simulink model "BD_PAR_AUTO_base_model"  (Simulink 10.3)
settings: Solver=ode1  StartTime=0.0  StopTime=max(cyc_mph(:,1))  FixedStep=1  MaxStep=1  RelTol=1e-3  AbsTol=1e-3
undefined symbols (not defined in the file): acc_dcdc_eff, acc_elec_eff, acc_elec_pwr, acc_mech_eff, acc_mech_pwr, acc_mech_trq, air_cp, amb_tmp, cs_charge_deplete_bool, cs_charge_trq, cs_electric_decel_spd, cs_electric_launch_spd_hi, cs_electric_launch_spd_lo, cs_hi_soc, cs_lo_soc, cs_min_trq_frac, cs_off_trq_frac, cyc_avg_time, cyc_cargo_mass, cyc_elevation_init, cyc_filter_bool, cyc_grade, cyc_mph, enable_sim_stop_distance, enable_sim_stop_max_spd, enable_sim_stop_speed, enable_sim_stop_time, enable_stop, enable_stop_fc, ess_cap_scale, ess_coulombic_eff, ess_init_soc, ess_max_ah_cap, ess_max_volts, ess_min_volts, ess_mod_airflow, ess_mod_cp, ess_mod_init_tmp, ess_module_mass, ess_module_num, ess_on, ess_r_chg, ess_r_dis, ess_res_scale_coef, ess_res_scale_fun, ess_set_tmp, ess_soc, ess_th_calc, ess_th_res_off, ess_th_res_on, ess_tmp, ess_voc, ex_calc, ex_cat_co_frac, ex_cat_ext_cp, ex_cat_ext_emisv, ex_cat_ext_init_tmp, ex_cat_ext_mass, ex_cat_ext_sarea, ex_cat_hc_frac ... (+168)
(part 4 of 15)

== system BD_PAR_AUTO_base_model/hydraulic torque converter for  parallel hybrid <htc>/effect of inertia (Nm) ==
  note: This block computes the torque required to overcome the inertia of the
      | turbine (plus 1/2 fluid in htc).
  turbine/output speed (rad/s) : Inport
  Constant : Constant  Value=htc_inertia
  Product : Product  SaturateOnIntegerOverflow=on
  d/dt : Derivative
  inertia torque (Nm) : Outport  InitialOutput=0
  wires:
  d/dt/1 -> Product/1
  turbine/output speed (rad/s)/1 -> d/dt/1
  Constant/1 -> Product/2
  Product/1 -> inertia torque (Nm)/1

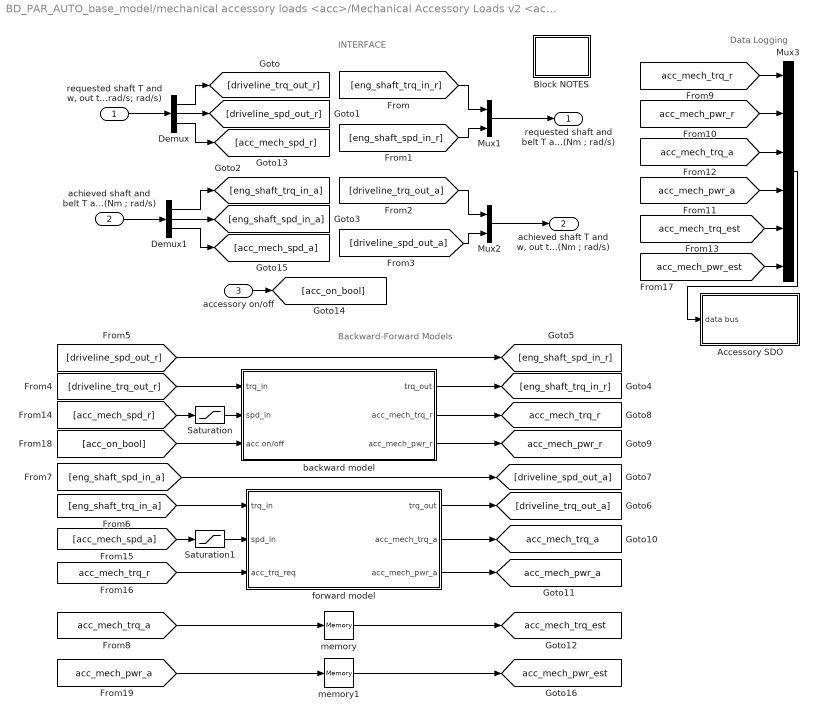
== system BD_PAR_AUTO_base_model/mechanical accessory loads <acc>/Mechanical Accessory Loads v2 <acc> ==
  note: Data Logging
  note: Backward-Forward Models
  note: INTERFACE
  "requested shaft T and w, out to the driveline  (Nm ; rad/s; rad/s)" : Inport
  "achieved shaft and belt T and w, in from the prime mover (Nm ; rad/s)" : Inport  Port=2
  accessory on/off : Inport  Port=3
  Accessory SDO : Subsystem
  Block NOTES : Subsystem
      mask Display: disp('Block\nNOTES')
  Demux : Demux  Outputs=3
      settings: DisplayOption=none
  Demux1 : Demux  Outputs=3
      settings: DisplayOption=none
  Mux1 : Mux  Inputs=2
  Mux2 : Mux  Inputs=2
  Mux3 : Mux  Inputs=6
  Saturation : Saturate  UpperLimit=acc_max_spd  LowerLimit=acc_min_spd
  Saturation1 : Saturate  UpperLimit=acc_max_spd  LowerLimit=acc_min_spd
  backward model : Subsystem
  forward model : Subsystem
  memory : Memory  InitialCondition=ic_mech_trq
  memory1 : Memory  InitialCondition=ic_mech_pwr
  "requested shaft and belt T and w, in from the prime mover (Nm ; rad/s)" : Outport
  "achieved shaft T and w, out to the driveline (Nm ; rad/s)" : Outport  Port=2
  tag scope: acc_mech_pwr_a=global, acc_mech_pwr_est=global, acc_mech_pwr_r=global, acc_mech_trq_a=global, acc_mech_trq_est=global, acc_mech_trq_r=global
  wires:
  [acc_mech_pwr_a] -> memory1/1
  [acc_mech_trq_a] -> memory/1
  memory1/1 -> [acc_mech_pwr_est]
  memory/1 -> [acc_mech_trq_est]
  [acc_mech_pwr_est] -> Mux3/6
  Demux/3 -> [acc_mech_spd_r]
  Demux1/3 -> [acc_mech_spd_a]
  [acc_mech_trq_r] -> forward model/3(acc_trq_req)
  Saturation/1 -> backward model/2(spd_in)
  [acc_mech_spd_r] -> Saturation/1
  Saturation1/1 -> forward model/2(spd_in)
  [acc_mech_spd_a] -> Saturation1/1
  forward model/3(acc_mech_pwr_a) -> [acc_mech_pwr_a]
  forward model/2(acc_mech_trq_a) -> [acc_mech_trq_a]
  forward model/1(trq_out) -> [driveline_trq_out_a]
  [acc_on_bool] -> backward model/3(acc on/off)
  accessory on/off/1 -> [acc_on_bool]
  [eng_shaft_trq_in_a] -> forward model/1(trq_in)
  [acc_mech_pwr_a] -> Mux3/4
  [acc_mech_trq_a] -> Mux3/3
  [eng_shaft_spd_in_a] -> [driveline_spd_out_a]
  [driveline_spd_out_r] -> [eng_shaft_spd_in_r]
  [acc_mech_trq_est] -> Mux3/5
  Mux3/1 -> Accessory SDO/1(data bus)
  [acc_mech_pwr_r] -> Mux3/2
  [acc_mech_trq_r] -> Mux3/1
  backward model/1(trq_out) -> [eng_shaft_trq_in_r]
  [driveline_trq_out_r] -> backward model/1(trq_in)
  backward model/3(acc_mech_pwr_r) -> [acc_mech_pwr_r]
  backward model/2(acc_mech_trq_r) -> [acc_mech_trq_r]
  [driveline_spd_out_a] -> Mux2/2
  [driveline_trq_out_a] -> Mux2/1
  Mux2/1 -> "achieved shaft T and w, out to the driveline (Nm ; rad/s)"/1
  [eng_shaft_spd_in_r] -> Mux1/2
  [eng_shaft_trq_in_r] -> Mux1/1
  Mux1/1 -> "requested shaft and belt T and w, in from the prime mover (Nm ; rad/s)"/1
  Demux1/2 -> [eng_shaft_spd_in_a]
  Demux1/1 -> [eng_shaft_trq_in_a]
  "achieved shaft and belt T and w, in from the prime mover (Nm ; rad/s)"/1 -> Demux1/1
  Demux/2 -> [driveline_spd_out_r]
  Demux/1 -> [driveline_trq_out_r]
  "requested shaft T and w, out to the driveline  (Nm ; rad/s; rad/s)"/1 -> Demux/1

== system BD_PAR_AUTO_base_model/motor/ controller <mc> par/Block NOTES ==
  note: Available torque is computed from available power by assuming that the ratio of rotor torque to input
      | (electric) power is the same for the actual/achievable situation as was computed for the request.  This
      | is mathematically equivalent to assuming that the motor/controller efficiency.  Rotor speed for the
      | actual/achievable calculations is as computed in the 'request' branch.
  note: This motor/controller model includes loss data, rotational inertia, and performance limits.

== system BD_PAR_AUTO_base_model/motor/ controller <mc> par/N-m drive torque per W input ==
  req'd input power (W) : Inport
  req'd rotor drive torque (Nm) : Inport  Port=2
  Block NOTES : Subsystem
      mask Display: disp('Block\nNOTES')
  Constant : Constant  Value=eps
  Constant1 : Constant  Value=0
  Constant2 : Constant  Value=inf
  Product : Product  Inputs=/*  SaturateOnIntegerOverflow=on
  Relational Operator : RelationalOperator  Operator=~=  RndMeth=Nearest  InputSameDT=on
  Sum : Sum  SaturateOnIntegerOverflow=on
  Switch : Switch  Threshold=eps
  Nm per W : Outport  InitialOutput=0
  wires:
  Constant2/1 -> Switch/3
  Constant1/1 -> Relational Operator/2
  req'd input power (W)/1 -> Relational Operator/1, Sum/2
  Sum/1 -> Product/1
  Switch/1 -> Nm per W/1
  Relational Operator/1 -> Switch/2
  Product/1 -> Switch/1
  req'd rotor drive torque (Nm)/1 -> Product/2
  Constant/1 -> Sum/1

== system BD_PAR_AUTO_base_model/motor/ controller <mc> par/documentation10 ==

== system BD_PAR_AUTO_base_model/motor/ controller <mc> par/effect of inertia (Nm) ==
  mc_spd_out_a : Inport
  Block NOTES : Subsystem
      mask Display: disp('Block\nNOTES')
  Constant : Constant  Value=eps
  Constant1 : Constant  Value=max(mc_max_trq)*mc_trq_scale*mc_overtrq_factor
  Constant2 : Constant  Value=gb_ratio(1)*fd_ratio/wh_radius
  Gain : Gain  Gain=mc_inertia  SaturateOnIntegerOverflow=on
  Memory : Memory
  MinMax : MinMax  Inputs=2
  Product : Product  SaturateOnIntegerOverflow=on
  Sum : Sum  SaturateOnIntegerOverflow=on
  Switch : Switch  Threshold=eps
  alpha : Derivative
  motor inertia as a function of total vehicle inertia (generous approximation) : Subsystem
  overall gear ratio / wh_radius : Product  Inputs=*/  SaturateOnIntegerOverflow=on
  out_1 : Outport  InitialOutput=0
  wires:
  Switch/1 -> overall gear ratio / wh_radius/2
  Constant2/1 -> Switch/3
  [veh_spd_a_rec] -> Switch/2, Sum/1
  Sum/1 -> Switch/1
  Constant/1 -> Sum/2
  motor inertia as a function of total vehicle inertia (generous approximation)/1(Out1) -> Product/2
  Memory/1 -> motor inertia as a function of total vehicle inertia (generous approximation)/1(gear ratio)
  Constant1/1 -> Product/1
  overall gear ratio / wh_radius/1 -> Memory/1
  Product/1 -> MinMax/2
  Gain/1 -> MinMax/1
  MinMax/1 -> out_1/1
  mc_spd_out_a/1 -> overall gear ratio / wh_radius/1, alpha/1
  alpha/1 -> Gain/1

== system BD_PAR_AUTO_base_model/motor/ controller <mc> par/enforce torque limit ==
  req'd motor torque (Nm) : Inport
  limited motor speed (rad/s) : Inport  Port=2
  Block NOTES : Subsystem
      mask Display: disp('Block\nNOTES')
  MinMax : MinMax  Inputs=2
  MinMax1 : MinMax  Function=max  Inputs=2
  Relational Operator2 : RelationalOperator  Operator=~=  RndMeth=Nearest  InputSameDT=on
  Switch : Switch
  To WS2 : ToWorkspace  VariableName=mc_max_trq_vec
      settings: MaxDataPoints=50000
  max gen torque : Lookup  InputValues=mc_map_spd*mc_spd_scale  Table=mc_max_gen_trq*mc_overtrq_factor*mc_trq_scale
  max torque : Lookup  InputValues=mc_map_spd*mc_spd_scale  Table=mc_max_trq*mc_overtrq_factor*mc_trq_scale
  limited motor torque (Nm) : Outport
  tag scope: mc_trq_limited=global
  wires:
  max gen torque/1 -> MinMax1/2
  limited motor speed (rad/s)/1 -> max gen torque/1, max torque/1
  Relational Operator2/1 -> [mc_trq_limited]
  MinMax/1 -> Switch/1
  MinMax1/1 -> Switch/3
  Switch/1 -> limited motor torque (Nm)/1, Relational Operator2/2
  req'd motor torque (Nm)/1 -> MinMax/1, MinMax1/1, Switch/2, Relational Operator2/1
  max torque/1 -> MinMax/2, To WS2/1

== system BD_PAR_AUTO_base_model/motor/ controller <mc> par/mc tmp ==
  Qmc_gen : Inport
  veh spd : Inport  Port=2
  key ON? : Inport  Port=3
  Enable : EnablePort  StatesWhenEnabling=reset
  1/mcp : Gain  Gain=1/(mc_mass*mc_cp)  SaturateOnIntegerOverflow=on
  >=0 : Saturate  UpperLimit=Inf  LowerLimit=0
  ">=0 " : Saturate  UpperLimit=Inf  LowerLimit=0
  Block NOTES : Subsystem
      mask Display: disp('Block\nNOTES')
  Mux10 : Mux  Inputs=2
  Mux9 : Mux  Inputs=2
  Qa : Fcn  Expr=u(1)*(mc_sarea*mc_trq_scale*mc_spd_scale)*u(2)
  Qc1 : Sum  Inputs=-+  SaturateOnIntegerOverflow=on
  Qnet : Sum  Inputs=+++  SaturateOnIntegerOverflow=on
  Qp2a,v7 : Fcn  Expr=amb_tmp-u(1)
  Qr : Fcn  Expr=0.9*(5.67e-8)*(mc_sarea*mc_trq_scale*mc_spd_scale)*((amb_tmp+273)^4 - (u(1)+273)^4)
  Tmc3 : Integrator  InitialCondition=mc_init_tmp
  Va/Vv : Gain  Gain=0.5  SaturateOnIntegerOverflow=on
  ha : Fcn  Expr=6 + 6*((abs(u(2))/1000))^0.25 + 60*(abs(u(1))/30)^0.63
  mc coolant : Subsystem  TreatAsAtomicUnit=on
  Tmc : Outport  InitialOutput=0
  Qmc_clt : Outport  Port=2  OutputWhenDisabled=reset  InitialOutput=0
  wires:
  Qnet/1 -> Qc1/2, mc coolant/2("Qmc ")
  Qc1/1 -> 1/mcp/1
  1/mcp/1 -> Tmc3/1
  Tmc3/1 -> Qp2a,v7/1, Qr/1, Tmc/1, mc coolant/1(Tcl)
  mc coolant/1(Qmc_clt) -> Qc1/1, >=0/1
  >=0/1 -> Qmc_clt/1
  key ON?/1 -> mc coolant/Enable
  veh spd/1 -> Va/Vv/1
  Qa/1 -> Qnet/2
  ">=0 "/1 -> Qnet/1
  Qmc_gen/1 -> ">=0 "/1
  Qr/1 -> Qnet/3
  Qp2a,v7/1 -> Mux10/2, Mux9/2
  ha/1 -> Mux10/1
  Va/Vv/1 -> Mux9/1
  Mux9/1 -> ha/1
  Mux10/1 -> Qa/1

== system BD_PAR_AUTO_base_model/motor/ controller <mc> par/motor controller logic interface ==
  w_mc_out_r : Inport
  P_mc_in_1lim : Inport  Port=2
  P_mc_in_r : Outport  InitialOutput=0
  tag scope: P_mc_in_1lim=global, w_mc_out_r=global
  wires:
  [P_mc_in_r] -> P_mc_in_r/1
  w_mc_out_r/1 -> [w_mc_out_r]
  P_mc_in_1lim/1 -> [P_mc_in_1lim]

== system BD_PAR_AUTO_base_model/motor/ controller <mc> par/motor speed estimator ==
  mc_spd_out_a : Inport
  <= max spd : Saturate  UpperLimit=max(mc_map_spd)*mc_spd_scale  LowerLimit=-inf
  Block NOTES : Subsystem
      mask Display: disp('Block\nNOTES')
  Constant : Constant  Value=eps
  Constant1 : Constant  Value=0
  Constant2 : Constant  Value=2
  Gain : Gain  Gain=0.447  SaturateOnIntegerOverflow=on
  Logical Operator1 : Logic
  Memory : Memory  InitialCondition=cyc_mph(1,2)*0.447/wh_radius*fd_ratio*max(gb_ratio)*tc_mc_to_fc_ratio
  Memory1 : Memory  InitialCondition=1
  Memory2 : Memory
  Product : Product  Inputs=**/  SaturateOnIntegerOverflow=on
  Relational : RelationalOperator  Operator=>  RndMeth=Nearest  InputSameDT=on
  Relational Operator1 : RelationalOperator  Operator=~=  RndMeth=Nearest  InputSameDT=on
  Sum : Sum  SaturateOnIntegerOverflow=on
  Sum1 : Sum  Inputs=-+  SaturateOnIntegerOverflow=on
  Switch : Switch  Threshold=eps
  Switch1 : Switch  Threshold=eps
  To Workspace7 : ToWorkspace  VariableName=mc_spd_est  SampleTime=-1
  Out1 : Outport
  tag scope: mc_spd_limited=global
  wires:
  Switch/1 -> Memory/1
  Memory1/1 -> Switch1/2
  Relational/1 -> Memory1/1
  Sum1/1 -> Relational/1
  Constant2/1 -> Relational/2
  [mpha] -> Sum1/1, Gain/1
  [cyc_mph_r] -> Sum1/2
  Constant/1 -> Sum/2
  Memory/1 -> Switch1/1
  Constant1/1 -> Switch/3
  [veh_spd_a_rec] -> Switch/2, Sum/1
  Gain/1 -> Product/2
  Sum/1 -> Product/3
  Product/1 -> Switch/1
  mc_spd_out_a/1 -> Product/1, Switch1/3
  Memory2/1 -> Logical Operator1/2
  Logical Operator1/1 -> [mc_spd_limited]
  Relational Operator1/1 -> Logical Operator1/1, Memory2/1
  Switch1/1 -> <= max spd/1, Relational Operator1/1
  <= max spd/1 -> Out1/1, To Workspace7/1, Relational Operator1/2

== system BD_PAR_AUTO_base_model/motor/ controller <mc> par/rotor drive torque available (Nm) ==
  torque per unit input power (N-m/W) : Inport
  available input power (W) : Inport  Port=2
  Block NOTES : Subsystem
      mask Display: disp('Block\nNOTES')
  Constant2 : Constant  Value=inf
  Constant3 : Constant  Value=0
  Product : Product  SaturateOnIntegerOverflow=on
  Relational Operator : RelationalOperator  Operator=~=  RndMeth=Nearest  InputSameDT=on
  Switch : Switch  Threshold=eps
  rotor drive torque available : Outport  InitialOutput=0
  wires:
  torque per unit input power (N-m/W)/1 -> Relational Operator/1, Product/1
  Switch/1 -> rotor drive torque available/1
  Relational Operator/1 -> Switch/2
  Product/1 -> Switch/1
  available input power (W)/1 -> Product/2
  Constant2/1 -> Relational Operator/2
  Constant3/1 -> Switch/3

== system BD_PAR_AUTO_base_model/power bus <pb>/Block NOTES ==
  note: This power bus requires power from (or distributes power to)
      | the generator first, taking the balance from the energy
      | storage system.

== system BD_PAR_AUTO_base_model/torque coupler <tc>/Block NOTES ==
  note: speed, while the motor's speed may be different.  The ratio of motor speed to main
      | output speed is stored in the variable tc_mc_to_fc_spd_ratio.
  note: This block models a chain- or belt-driven torque coupler, with three gears:  one each
      | for the motor, main input (the engine or gearbox), and main output (to the gearbox
      | or final drive).  It includes losses in the chain or belt, but leaves inertia effects to be
      | considered in the appropriate component.
      |
      | The entire torque required out of the torque coupler (plus losses) is required from the
      | engine.  The engine provides only as much torque as its engine controller (see the
      | <vc> block) allows.  Any remaining unmet torque request is submitted to the motor,
      | which meets the request to the best of its ability.
      |
      | The torque converter output speed is limited by the maximum speeds of both the
      | motor and the engine.
      |
      | The loss torque is zero when the gears are not turning, and is applied at the output
      |  gear.
      |
      | The gears connecting the main input and main output to the torque converter's belt
      | or chain are assumed to be of the same size, so that main input speed = main output

== system BD_PAR_AUTO_base_model/torque coupler <tc>/help ==

== system BD_PAR_AUTO_base_model/torque coupler <tc>/loss (Nm) ==
  note: The loss torque is zero when the gears are not turning,
      | and is applied at the torque coupler's output gear.
  tc output speed (rad/s) : Inport
  Constant : Constant  Value=0
  Switch : Switch  Threshold=eps
  torque coupler loss torque (Nm) : Constant  Value=tc_loss
  drag torque (Nm) : Outport  InitialOutput=0
  wires:
  torque coupler loss torque (Nm)/1 -> Switch/1
  Switch/1 -> drag torque (Nm)/1
  tc output speed (rad/s)/1 -> Switch/2
  Constant/1 -> Switch/3

== system BD_PAR_AUTO_base_model/vehicle <veh>/Block NOTES ==
  note: A slight simplification, the assumption that (speed_at_end_of_time_step)^2 is roughly equal to
      | (speed_at_end_of_time_step)*(speed_at_beginning_of_time_step), is used to avoid solving
      | a quadratic equation in the solution of v=v(Ftract).
  note: This block uses the required vehicle speed with vehicle parameters and the previous speed
      | and classic, straightforward equations to determine the tractive force required at the tire/road interface.
  note: If no drivetrain component ran up against its performance limit during the time step, the achieved speed
      | is taken to be the requested speed.
  note: Given the tractive force available, this block uses the same equations to determine the achievable speed.

== system BD_PAR_AUTO_base_model/vehicle <veh>/force req'd to accelerate (N) ==
  v(m/s) : Inport
  v prev : Inport  Port=2
  Clock : Clock
  Memory : Memory  InitialCondition=-0.1
  Product1 : Product  Inputs=**/  SaturateOnIntegerOverflow=on
  Sum : Sum  Inputs=+-  SaturateOnIntegerOverflow=on
  Sum1 : Sum  Inputs=+-  SaturateOnIntegerOverflow=on
  current veh mass : Subsystem
  (N) : Outport  InitialOutput=0
  wires:
  current veh mass/1(Out1) -> Product1/1
  Clock/1 -> Sum1/1, Memory/1
  Memory/1 -> Sum1/2
  Product1/1 -> (N)/1
  v prev/1 -> Sum/2
  v(m/s)/1 -> Sum/1
  Sum1/1 -> Product1/3
  Sum/1 -> Product1/2

== system BD_PAR_AUTO_base_model/vehicle <veh>/force req'd to ascend (N) ==
  average vehicle speed over time step (m/s) : Inport
  Constant : Constant  Value=veh_gravity
  Constant1 : Constant  Value=0
  Product : Product  Inputs=3  SaturateOnIntegerOverflow=on
  Switch : Switch
  Trigonometric Function : Trigonometry  Operator=atan
  Trigonometric Function1 : Trigonometry
  current veh mass : Subsystem
  (N) : Outport  InitialOutput=0
  wires:
  current veh mass/1(Out1) -> Product/3
  average vehicle speed over time step (m/s)/1 -> Switch/2
  Constant1/1 -> Switch/3
  Switch/1 -> (N)/1
  Product/1 -> Switch/1
  Constant/1 -> Product/1
  [grade] -> Trigonometric Function/1
  Trigonometric Function1/1 -> Product/2
  Trigonometric Function/1 -> Trigonometric Function1/1

== system BD_PAR_AUTO_base_model/vehicle <veh>/force req'd to overcome aerodynamic drag (N) ==
  average vehicle speed over time step (m/s) : Inport
  Constant : Constant  Value=veh_air_density*veh_CD*veh_FA*0.5
  Product : Product  Inputs=3  SaturateOnIntegerOverflow=on
  D aero(N) : Outport  InitialOutput=0
  wires:
  Product/1 -> D aero(N)/1
  Constant/1 -> Product/3
  average vehicle speed over time step (m/s)/1 -> Product/2, Product/1

== system BD_PAR_AUTO_base_model/vehicle <veh>/help ==

== system BD_PAR_AUTO_base_model/vehicle <veh>/record achieved force outputs ==
  spd_prev : Inport
  spd : Inport  Port=2
  Gain1 : Gain  Gain=0.5  SaturateOnIntegerOverflow=on
  Product{,1..3} (4 alike) : Product  SaturateOnIntegerOverflow=on
  Sum2 : Sum  SaturateOnIntegerOverflow=on
  To Workspace1 : ToWorkspace  VariableName=veh_pwr_rr_a  SampleTime=-1
  To Workspace4 : ToWorkspace  VariableName=veh_pwr_accel_a  SampleTime=-1
  To Workspace6 : ToWorkspace  VariableName=veh_pwr_drag_a  SampleTime=-1
  To Workspace7 : ToWorkspace  VariableName=veh_pwr_ascent_a  SampleTime=-1
  force req'd to accelerate (N)1 : Subsystem
  force req'd to ascend (N)1 : Subsystem
  force req'd to overcome aerodynamic drag (N)1 : Subsystem
  rolling resistance force : Subsystem  BlockChoice=force req'd to overcome rolling resistance (N)
      settings: AttributesFormatString=%<BlockChoice>  TemplateBlock=lib_vehicle/Submodels/rolling resistance force  MemberBlocks=force req'd to overcome rolling resistance (N),force req'd to overcome rolling resistance (N) j2452
  tag scope: veh_pwr_accel_a=global, veh_pwr_ascent_a=global, veh_pwr_drag_a=global, veh_pwr_rr_a=global
  wires:
  Gain1/1 -> [vel_ave], rolling resistance force/1(average vehicle speed over time step (m/s)), force req'd to ascend (N)1/1(average vehicle speed over time step (m/s)), force req'd to overcome aerodynamic drag (N)1/1(average vehicle speed over time step (m/s))
  Product3/1 -> To Workspace1/1, [veh_pwr_rr_a]
  [vel_ave] -> Product3/2
  Product2/1 -> [veh_pwr_ascent_a], To Workspace7/1
  [vel_ave] -> Product2/2
  [vel_ave] -> Product1/2
  [vel_ave] -> Product/2
  Product1/1 -> [veh_pwr_drag_a], To Workspace6/1
  Product/1 -> [veh_pwr_accel_a], To Workspace4/1
  force req'd to accelerate (N)1/1((N)) -> Product/1
  rolling resistance force/1(Fr (N)) -> Product3/1
  force req'd to ascend (N)1/1((N)) -> Product2/1
  force req'd to overcome aerodynamic drag (N)1/1(D aero(N)) -> Product1/1
  spd_prev/1 -> Sum2/2, force req'd to accelerate (N)1/2(v prev)
  spd/1 -> Sum2/1, force req'd to accelerate (N)1/1(v(m/s))
  Sum2/1 -> Gain1/1

== system BD_PAR_AUTO_base_model/vehicle <veh>/rolling resistance force ==
  average vehicle speed over time step (m/s) : Inport
  force req'd to overcome rolling resistance (N) : Subsystem
  Fr (N) : Outport
  wires:
  average vehicle speed over time step (m/s)/1 -> force req'd to overcome rolling resistance (N)/1(average vehicle speed over time step (m/s))
  force req'd to overcome rolling resistance (N)/1(Fr (N)) -> Fr (N)/1

== system BD_PAR_AUTO_base_model/vehicle <veh>/vehicle speed ==
  vehicle speed at beginning of time step (m/s) : Inport
  "available tractive force and linear speed (N), (m/s)" : Inport  Port=2
  vehicle speed (m/s) : Subsystem
  vehicle speed achievable at end of time step (m/s) : Outport
  wires:
  vehicle speed at beginning of time step (m/s)/1 -> vehicle speed (m/s)/1(vehicle speed at beginning of time step (m/s))
  "available tractive force and linear speed (N), (m/s)"/1 -> vehicle speed (m/s)/2("available tractive force and linear speed (N), (m/s)")
  vehicle speed (m/s)/1(vehicle speed achievable at end of time step (m/s)) -> vehicle speed achievable at end of time step (m/s)/1

== system BD_PAR_AUTO_base_model/wheel and axle  front/rear <wh>/Block NOTES ==
  note: This block determines the required axle torque and speed given the tractive force and
      | speed required to meet the trace in the top blocks, and determines the available tractive
      | force and possible vehicle speed given the drivetrain-input torque and rotational speed
      | in the bottom blocks.  The "wheel control" blocks apply the braking strategy and ensure
      | that accelerations beyond the capability of the tires are not requested.

== system BD_PAR_AUTO_base_model/wheel and axle  front/rear <wh>/effect of  inertia (Nm) ==
  note: This block computes the torque required to overcome the inertia of the
      | wheels and axle.
  axle input speed (rad/s) : Inport
  Constant : Constant  Value=wh_inertia
  Product : Product  SaturateOnIntegerOverflow=on
  d/dt : Derivative
  inertia torque (Nm) : Outport  InitialOutput=0
  wires:
  Product/1 -> inertia torque (Nm)/1
  Constant/1 -> Product/2
  axle input speed (rad/s)/1 -> d/dt/1
  d/dt/1 -> Product/1

== system BD_PAR_AUTO_base_model/wheel and axle  front/rear <wh>/front brake ==
  F_brake : Inport
  Constant : Constant  Value=wh_max_front_brake_force
  Terminator : Terminator
  F_brake_max : Outport  InitialOutput=0
  wires:
  Constant/1 -> F_brake_max/1
  F_brake/1 -> Terminator/1

== system BD_PAR_AUTO_base_model/wheel and axle  front/rear <wh>/front force ==
  In1 : Inport
  In2 : Inport  Port=2
  Product1 : Product  SaturateOnIntegerOverflow=on
  Sum2 : Sum  Inputs=-+  SaturateOnIntegerOverflow=on
  To Workspace12 : ToWorkspace  VariableName=wh_front_brake_r  SampleTime=-1
  brake request  controller interface : Subsystem
  tractive torque req/d of drivetrain (Nm) : Gain  Gain=wh_radius  SaturateOnIntegerOverflow=on
  Out1 : Outport
  wires:
  tractive torque req/d of drivetrain (Nm)/1 -> Out1/1
  In2/1 -> Product1/2
  In1/1 -> Product1/1
  Product1/1 -> Sum2/2
  Sum2/1 -> tractive torque req/d of drivetrain (Nm)/1
  brake request  controller interface/1(F_front_brake_req) -> To Workspace12/1, Sum2/1

== system BD_PAR_AUTO_base_model/wheel and axle  front/rear <wh>/front/rear brake controller interface (achievable) ==
  F_drivetrain_ach : Inport
  w_wheel_ach : Inport  Port=2
  F_rear_drivetrain_ach : Inport  Port=3
  F_max_front_brake : Inport  Port=4
  F_max_rear_brake : Inport  Port=5
  F_front_brake : Outport  InitialOutput=0
  F_rear_brake : Outport  Port=2  InitialOutput=0
  tag scope: F_drivetrain_ach=global, F_max_front_brake=global, F_max_rear_brake=global, F_rear_drivetrain_ach=global, w_wheel_ach=global
  wires:
  F_rear_drivetrain_ach/1 -> [F_rear_drivetrain_ach]
  F_max_rear_brake/1 -> [F_max_rear_brake]
  F_max_front_brake/1 -> [F_max_front_brake]
  F_drivetrain_ach/1 -> [F_drivetrain_ach]
  w_wheel_ach/1 -> [w_wheel_ach]
  [F_front_brake] -> F_front_brake/1
  [F_rear_brake] -> F_rear_brake/1

== system BD_PAR_AUTO_base_model/wheel and axle  front/rear <wh>/help ==

== system BD_PAR_AUTO_base_model/wheel and axle  front/rear <wh>/limits and losses diagnostics ==
  speed : Inport
  front brake : Inport  Port=2
  front brake max : Inport  Port=3
  rear brake max : Inport  Port=4
  rear brake : Inport  Port=5
  Gain : Gain  Gain=-1  SaturateOnIntegerOverflow=on
  Logical Operator : Logic  Operator=OR
  Product : Product  SaturateOnIntegerOverflow=on
  Relational Operator1 : RelationalOperator  Operator===  RndMeth=Nearest  InputSameDT=on
  Relational Operator2 : RelationalOperator  Operator===  RndMeth=Nearest  InputSameDT=on
  Sum3 : Sum  SaturateOnIntegerOverflow=on
  To Workspace6 : ToWorkspace  VariableName=wh_brake_loss_pwr  SampleTime=-1
  tag scope: brake_limited=global
  wires:
  rear brake/1 -> Relational Operator2/2, Sum3/2
  rear brake max/1 -> Relational Operator2/1
  front brake max/1 -> Relational Operator1/2
  front brake/1 -> Relational Operator1/1, Sum3/1
  speed/1 -> Product/1
  Relational Operator2/1 -> Logical Operator/2
  Relational Operator1/1 -> Logical Operator/1
  Logical Operator/1 -> [brake_limited]
  Product/1 -> To Workspace6/1
  Sum3/1 -> Gain/1
  Gain/1 -> Product/2

== system BD_PAR_AUTO_base_model/wheel and axle  front/rear <wh>/loss (Nm) ==
  note: The loss torque is zero when the axle is not turning.
  axle speed (rad/s) : Inport
  Constant : Constant  Value=0
  Switch : Switch  Threshold=eps
  veh mass calc : Subsystem
  wheel & axle bearing drag (Nm) : Lookup  InputValues=wh_axle_loss_mass  Table=wh_axle_loss_trq
  drag torque (Nm) : Outport  InitialOutput=0
  wires:
  wheel & axle bearing drag (Nm)/1 -> Switch/1
  Constant/1 -> Switch/3
  axle speed (rad/s)/1 -> Switch/2
  Switch/1 -> drag torque (Nm)/1
  veh mass calc/1(Out1) -> wheel & axle bearing drag (Nm)/1

== system BD_PAR_AUTO_base_model/wheel and axle  front/rear <wh>/rear brake ==
  F_brake : Inport
  Constant : Constant  Value=wh_max_rear_brake_force
  Terminator : Terminator
  F_brake_max : Outport  InitialOutput=0
  wires:
  F_brake/1 -> Terminator/1
  Constant/1 -> F_brake_max/1

== system BD_PAR_AUTO_base_model/wheel and axle  front/rear <wh>/rear force ==
  In1 : Inport
  In2 : Inport  Port=2
  Product2 : Product  SaturateOnIntegerOverflow=on
  Sum1 : Sum  Inputs=-+  SaturateOnIntegerOverflow=on
  Sum4 : Sum  Inputs=-+  SaturateOnIntegerOverflow=on
  To Workspace12 : ToWorkspace  VariableName=wh_rear_brake_r  SampleTime=-1
  brake request controller interface1 : Subsystem
  tractive torque req/d of drivetrain (Nm)1 : Gain  Gain=wh_radius  SaturateOnIntegerOverflow=on
  Out1 : Outport
  wires:
  Sum1/1 -> Sum4/2
  Product2/1 -> Sum1/1
  In2/1 -> Product2/2
  In1/1 -> Sum1/2, Product2/1
  tractive torque req/d of drivetrain (Nm)1/1 -> Out1/1
  Sum4/1 -> tractive torque req/d of drivetrain (Nm)1/1
  brake request controller interface1/1(F_rear_brake_req) -> To Workspace12/1, Sum4/1

== system BD_PAR_AUTO_base_model/wheel and axle  front/rear <wh>/tire slip model (m/s) ==
  note: See note regarding sum in backward path
  weight borne  by front axle (N) : Inport
  total tractive  force available (N) : Inport  Port=2
  axle speed available (rad/s) : Inport  Port=3
  axle speed req'd (rad/s) : Inport  Port=4
  vehicle speed required (m/s) : Inport  Port=5
  weight borne by  rear axle (N) : Inport  Port=6
  front fraction : Inport  Port=7
  Abs1 : Abs
  Block NOTES : Subsystem
      mask Display: disp('Block\nNOTES')
  Constant : Constant  Value=1e-3
  Constant5 : Constant
  Constant6 : Constant  Value=wh_radius
  Fcn : Fcn  Expr=1/u
  Relational Operator1 : RelationalOperator  Operator=>  RndMeth=Nearest  InputSameDT=on
  Sum1 : Sum  Inputs=+-  SaturateOnIntegerOverflow=on
  Sum2 : Sum  SaturateOnIntegerOverflow=on
  Sum3 : Sum  SaturateOnIntegerOverflow=on
  Sum4 : Sum  Inputs=-+  SaturateOnIntegerOverflow=on
  Switch1 : Switch  Threshold=eps
  front axle : Subsystem
  front frac : Product  SaturateOnIntegerOverflow=on
  rear axle : Subsystem
  vehicle speed (m/s) : Product  Inputs=3  SaturateOnIntegerOverflow=on
  possible vehicle speed (m/s) : Outport  InitialOutput=0
  tag scope: veh_spd_a_rec=global
  wires:
  Sum2/1 -> Sum3/1
  rear axle/1(Out1) -> Sum2/2
  front axle/1(Out1) -> Sum2/1
  Sum1/1 -> rear axle/2(In2)
  front frac/1 -> Sum1/2, front axle/2(In2)
  front fraction/1 -> front frac/2
  total tractive  force available (N)/1 -> Sum1/1, front frac/1
  weight borne by  rear axle (N)/1 -> rear axle/1(In1)
  vehicle speed (m/s)/1 -> [veh_spd_a_rec], Switch1/1
  Switch1/1 -> possible vehicle speed (m/s)/1
  weight borne  by front axle (N)/1 -> front axle/1(In1)
  Abs1/1 -> Relational Operator1/1
  Constant/1 -> Relational Operator1/2
  axle speed req'd (rad/s)/1 -> Sum4/2
  Sum4/1 -> Abs1/1
  vehicle speed required (m/s)/1 -> Switch1/3
  Relational Operator1/1 -> Switch1/2
  Constant6/1 -> vehicle speed (m/s)/3
  axle speed available (rad/s)/1 -> vehicle speed (m/s)/2, Sum4/1
  Constant5/1 -> Sum3/2
  Fcn/1 -> vehicle speed (m/s)/1
  Sum3/1 -> Fcn/1

== system BD_PAR_AUTO_base_model/wheel and axle  front/rear <wh>/tire slip model (rad/s) ==
  note: Question: for front and rear, is it the sum of or min/max? tm:020703
  note: This block implements the effects of finite tire slip
      | (with respect to the road) on the vehicle speed/wheel speed relationship.
  note: Slip is defined as s=(omega*r - v) / v.  The one-to-one mapping of slip to normalized
      | tractive force, F_tract/W_front_axle, up to the maximum, is stored in the variables
      | "wh_slip" and "wh_slip_force_coeff."
  total tractive  force requested (N) : Inport
  requested time-step average vehicle speed (m/s) : Inport  Port=2
  weight borne by front axle (N) : Inport  Port=3
  weight borne by  rear axle (N)1 : Inport  Port=4
  front traction ratio : Inport  Port=5
  Constant5 : Constant
  Constant6 : Constant  Value=1/wh_radius
  Sum1 : Sum  Inputs=+-  SaturateOnIntegerOverflow=on
  Sum2 : Sum  SaturateOnIntegerOverflow=on
  Sum3 : Sum  SaturateOnIntegerOverflow=on
  To Workspace6 : ToWorkspace  VariableName=wh_slip_r  SampleTime=-1
  front frac : Product  SaturateOnIntegerOverflow=on
  front slip : Subsystem
  rear slip : Subsystem
  wheel speed (rad/s) : Product  Inputs=3  SaturateOnIntegerOverflow=on
  slip-augmented rotational speed (rad/s) : Outport  InitialOutput=0
  wires:
  Sum2/1 -> To Workspace6/1, Sum3/1
  rear slip/1(Out1) -> Sum2/2
  front slip/1(Out1) -> Sum2/1
  weight borne by  rear axle (N)1/1 -> rear slip/1(In1)
  Sum1/1 -> rear slip/2(In2)
  front traction ratio/1 -> front frac/2
  total tractive  force requested (N)/1 -> Sum1/1, front frac/1
  front frac/1 -> front slip/2(In2), Sum1/2
  wheel speed (rad/s)/1 -> slip-augmented rotational speed (rad/s)/1
  Constant5/1 -> Sum3/2
  Sum3/1 -> wheel speed (rad/s)/2
  Constant6/1 -> wheel speed (rad/s)/3
  requested time-step average vehicle speed (m/s)/1 -> wheel speed (rad/s)/1
  weight borne by front axle (N)/1 -> front slip/1(In1)

== system BD_PAR_AUTO_base_model/wheel and axle  front/rear <wh>/traction controller interface ==
  F_req : Inport
  v_ave_req : Inport  Port=2
  F_req_limited : Outport  InitialOutput=0
  v_req_limited : Outport  Port=2  InitialOutput=0
  wt_front_axle : Outport  Port=3  InitialOutput=0
  wt_rear_axle : Outport  Port=4  InitialOutput=0
  front_traction_ratio : Outport  Port=5  InitialOutput=0
  tag scope: F_req=global, v_ave_req=global
  wires:
  [front_traction_ratio] -> front_traction_ratio/1
  [wt_rear_axle] -> wt_rear_axle/1
  v_ave_req/1 -> [v_ave_req]
  F_req/1 -> [F_req]
  [wt_front_axle] -> wt_front_axle/1
  [v_req_limited] -> v_req_limited/1
  [F_req_limited] -> F_req_limited/1

== system BD_PAR_AUTO_base_model/<vc> par auto/braking strategy/Block NOTES ==
  note: This controller determines how much braking
      | force the front and rear  friction brakes will supply.

== system BD_PAR_AUTO_base_model/<vc> par auto/config traction control/traction control 2 axle ==
  time-average vehicle speed  req'd (m/s) : Inport
  vehicle speed at beginning of time  step (m/s) : Inport  Port=2
  total tractive force req'd (N) : Inport  Port=3
  Block NOTES : Subsystem
      mask Display: disp('Block\nNOTES')
  apply tire traction limit to req'd speed (m/s) : Subsystem
  enforce max.  front axle tractive force  due to slip (N) : Subsystem
  req'd force (N) : Outport  InitialOutput=0
  req'd speed (m/s) : Outport  Port=2  InitialOutput=0
  weight on front axle (N) : Outport  Port=3  InitialOutput=0
  weight on rear axle (N) : Outport  Port=4  InitialOutput=0
  front/total  traction ratio : Outport  Port=5  InitialOutput=0
  wires:
  enforce max.  front axle tractive force  due to slip (N)/4(front/total traction ratio) -> front/total  traction ratio/1
  enforce max.  front axle tractive force  due to slip (N)/3(weight on rear axle (N)) -> weight on rear axle (N)/1
  time-average vehicle speed  req'd (m/s)/1 -> apply tire traction limit to req'd speed (m/s)/1("requested time-step  average vehicle speed (m/s) ")
  vehicle speed at beginning of time  step (m/s)/1 -> apply tire traction limit to req'd speed (m/s)/2(vehicle speed at beginning of time step (m/s)), enforce max.  front axle tractive force  due to slip (N)/3(speed at beginning of time step (m/s))
  enforce max.  front axle tractive force  due to slip (N)/2(weight on front axle (N)) -> weight on front axle (N)/1
  enforce max.  front axle tractive force  due to slip (N)/1(slip-limited force (N)) -> req'd force (N)/1
  total tractive force req'd (N)/1 -> enforce max.  front axle tractive force  due to slip (N)/1(tractive force req'd at tire/road interface (N))
  apply tire traction limit to req'd speed (m/s)/1(out_1) -> req'd speed (m/s)/1, enforce max.  front axle tractive force  due to slip (N)/2(requested time-step average vehicle speed (m/s))

== system BD_PAR_AUTO_base_model/<vc> par auto/engine on (parallel hybrid)/Block NOTES1 ==
  note: This engine state computer keeps the engine on if:
      | [
      | 1) key is on, AND
      | 2) (trq is too high AND speed is too high for idle) OR engine is allowed to idle, AND
      | 3) vehicle speed >= cs_electric_launch_spd [ in m/s ], AND
      | 4) req'd trq > (cs_off_trq_frac * max_trq_at_spd) OR SOC<cs_lo_soc
      | ]
      | OR
      | [ engine was previously on AND the transmission is shifting ]
      |
      | The last condition is added to prevent the engine from unrealistically
      | shutting down for a second or two during a shift.

== system BD_PAR_AUTO_base_model/<vc> par auto/engine on (parallel hybrid)/Subsystem ==
  in_1 : Inport
  Clock : Clock
  Constant1 : Constant  Value=n
  Constant2 : Constant
  Integrator : Integrator
  Memory : Memory  InitialCondition=-0.1
  Memory1 : Memory
  Product : Product  Inputs=*/  InputSameDT=on  RndMeth=Zero  SaturateOnIntegerOverflow=on  OutDataTypeStr=Inherit: Same as first input
  Product1 : Product  InputSameDT=on  RndMeth=Zero  SaturateOnIntegerOverflow=on  OutDataTypeStr=Inherit: Same as first input
  Relational Operator : RelationalOperator  Operator=<=  RndMeth=Nearest  InputSameDT=on
  Sum : Sum  Inputs=+-  InputSameDT=on  SaturateOnIntegerOverflow=on  OutDataTypeStr=Inherit: Same as first input
  Sum1 : Sum  Inputs=|+-  InputSameDT=on  SaturateOnIntegerOverflow=on  OutDataTypeStr=Inherit: Same as first input
  Switch{,1..3} (4 alike) : Switch  Threshold=eps
  Variable Transport Delay : VariableTransportDelay  MaximumDelay=n
  out_1 : Outport  InitialOutput=0
  wires:
  Product/1 -> out_1/1
  Sum/1 -> Product/1
  Variable Transport Delay/1 -> Sum/2
  Integrator/1 -> Variable Transport Delay/1, Sum/1
  Relational Operator/1 -> Switch/2
  Constant1/1 -> Product1/2
  Clock/1 -> Sum1/1, Memory/1, Relational Operator/1, Switch/1
  Memory/1 -> Sum1/2
  Sum1/1 -> Product1/1
  Product1/1 -> Relational Operator/2, Switch/3
  Switch/1 -> Variable Transport Delay/2, Switch1/2, Switch1/1
  Constant2/1 -> Switch1/3
  Switch1/1 -> Product/2
  Switch2/1 -> Integrator/1
  Switch3/1 -> Memory1/1
  in_1/1 -> Switch2/3, Switch3/3
  Memory1/1 -> Switch2/1, Switch3/1
  [shifting] -> Switch2/2, Switch3/2

== system BD_PAR_AUTO_base_model/<vc> par auto/engine on (parallel hybrid)/key_on ==
  Clock : Clock
  Fcn1 : Fcn  Expr=rem(u[1],period)
  Look-Up Table : Lookup  InputValues=t  Table=y
  out_1 : Outport  InitialOutput=0
  wires:
  Fcn1/1 -> Look-Up Table/1
  Clock/1 -> Fcn1/1
  Look-Up Table/1 -> out_1/1

== system BD_PAR_AUTO_base_model/<vc> par auto/engine on (parallel hybrid)/repeated cycle:  speed required at end of NEXT step ==
  Clock : Clock
  Fcn1 : Fcn  Expr=rem(u[1],period)
  Look-Up Table : Lookup  InputValues=t  Table=y
  Memory : Memory  InitialCondition=-0.1
  Sum : Sum  Inputs=+-  InputSameDT=on  SaturateOnIntegerOverflow=on  OutDataTypeStr=Inherit: Same as first input
  Sum1 : Sum  InputSameDT=on  SaturateOnIntegerOverflow=on  OutDataTypeStr=Inherit: Same as first input
  out_1 : Outport  InitialOutput=0
  wires:
  Sum1/1 -> Look-Up Table/1
  Look-Up Table/1 -> out_1/1
  Fcn1/1 -> Sum1/1
  Sum/1 -> Sum1/2
  Memory/1 -> Sum/2
  Clock/1 -> Fcn1/1, Memory/1, Sum/1

== system BD_PAR_AUTO_base_model/<vc> par auto/front and rear brake controller (achievable)/Block NOTES ==
  note: This block apportions required friction braking force between the
      | front (drive) and rear brakes.  Vehicle speed for brake strategy is
      | computed assuming zero slip.

== system BD_PAR_AUTO_base_model/<vc> par auto/front and rear brake controller (achievable)/braking force supplied by front friction brakes (N) ==
  add'l braking force req'd (N) : Inport
  possible speed (mph) : Inport  Port=2
  max front brake force (N) : Inport  Port=3
  Block NOTES : Subsystem
      mask Display: disp('Block\nNOTES')
  Constant : Constant  Value=1+eps
  Constant1 : Constant  Value=0.6
  Keep 0<frac<1 : Saturate  UpperLimit=1  LowerLimit=0
  MinMax : MinMax  Function=max  Inputs=2  InputSameDT=on  SaturateOnIntegerOverflow=on
  Product : Product  Inputs=**  InputSameDT=on  RndMeth=Zero  SaturateOnIntegerOverflow=on  OutDataTypeStr=Inherit: Same as first input
  Product1 : Product  Inputs=*/  InputSameDT=on  RndMeth=Zero  SaturateOnIntegerOverflow=on  OutDataTypeStr=Inherit: Same as first input
  Saturation : Saturate  UpperLimit=max(wh_fa_fric_brake_mph)  LowerLimit=min(wh_fa_fric_brake_mph)
  Saturation1 : Saturate  UpperLimit=max(wh_fa_dl_brake_mph)  LowerLimit=min(wh_fa_dl_brake_mph)
  Sum : Sum  Inputs=-+  InputSameDT=on  SaturateOnIntegerOverflow=on  OutDataTypeStr=Inherit: Same as first input
  Switch1 : Switch  Threshold=eps
  driveline braking fraction : Lookup  InputValues=wh_fa_dl_brake_mph  Table=wh_fa_dl_brake_frac
  front friction braking fraction : Lookup  InputValues=wh_fa_fric_brake_mph  Table=wh_fa_fric_brake_frac
  braking force from front-axle friction brakes (N) : Outport  InitialOutput=0
  wires:
  possible speed (mph)/1 -> Saturation/1, Saturation1/1
  Saturation1/1 -> driveline braking fraction/1
  Saturation/1 -> front friction braking fraction/1
  Constant1/1 -> Switch1/3
  Sum/1 -> Switch1/2, Product1/2
  Product1/1 -> Switch1/1
  front friction braking fraction/1 -> Product1/1
  driveline braking fraction/1 -> Sum/1
  Constant/1 -> Sum/2
  add'l braking force req'd (N)/1 -> Product/1
  max front brake force (N)/1 -> MinMax/2
  Product/1 -> MinMax/1
  MinMax/1 -> braking force from front-axle friction brakes (N)/1
  Switch1/1 -> Keep 0<frac<1/1
  Keep 0<frac<1/1 -> Product/2

== system BD_PAR_AUTO_base_model/<vc> par auto/gearbox control for use w/ AT/Block NOTES ==
  note: This gearbox control block computes the current gear number given the gearbox's
      | req'd output torque and speed and an estimate its efficiency.  Upshifts occur, given a
      | certain engine speed,  when the estimated engine load falls below the upshift curve
      | in engine speed/load space, and downshifts likewise occur when estimated engine
      | load rises above the downshift curve.  Separate upshift and downshift curves are
      | defined for each gear.  An upshift may not be immediately followed by a downshift.
      | If the tires are about to slip, don't upshift unless the engine would be at max. speed.
      | Enforce this rule by setting the load to 1 when the tires are about to slip.
  note: Lock-up of the HTC occurs when it is supposed to for the current gear, AND
      | the transmission isn't shifting, AND
      | the lockup wouldn't precipitate an immediate downshift.

== system BD_PAR_AUTO_base_model/<vc> par auto/gearbox control for use w/ AT/Speed Dependent Shifting ==
  note: storing shifting and gear ratio
      | information to workspace
  note: decel case
  note: accel case
  note: accel
      | case
  note: decel
      | case
  note: delta speed
  note: SPEED
      | DEPENDENT
      | SHIFT
      | SIGNAL
  "velocity required (limited) " : Inport
  Look-Up Table (gear for downshift) : Lookup  InputValues="tx_spd_dep_dnshift(:,1)   % vector of speeds m/s"  Table="tx_spd_dep_dnshift(:,2)  % gear number--must be step function"
  Look-Up Table (gear for upshift) : Lookup  InputValues="tx_spd_dep_upshift(:,1)   % vector of speeds in m/s"  Table="tx_spd_dep_upshift(:,2)  % gear number--must be step function"
  Mux : Mux  Inputs=2
  Mux2 : Mux  Inputs=2
  New gear ratio : ToWorkspace  VariableName=new_gear_ratio
      settings: MaxDataPoints=50000
  Rounding Function : Rounding  Operator=round
  Rounding Function1 : Rounding  Operator=round
  Saturation4 : Saturate  UpperLimit=gb_gears_num  LowerLimit=1
  Saturation5 : Saturate  UpperLimit=gb_gears_num  LowerLimit=1
  "delta speed (\"+\" is acceleration)" : Sum  Inputs=-+  InputSameDT=on  SaturateOnIntegerOverflow=on  OutDataTypeStr=Inherit: Same as first input
  gear ratio6 : Lookup  InputValues=[1:length(gb_ratio)]  Table=gb_ratio
  gear ratio8 : Lookup  InputValues=[1:length(gb_ratio)]  Table=gb_ratio
  prev veh speed : Memory  InitialCondition=1
  shifting : Subsystem
  shifting1 : Subsystem
  switch for gear number : Switch  Threshold=eps
  switch for gear ratio and shifting (muxed) : Switch  Threshold=eps
  total fuel used (gal) : ToWorkspace  VariableName=neg_gear_num
      settings: MaxDataPoints=50000
  gear ratio and shifting : Outport
  gear number : Outport  Port=2
  wires:
  Rounding Function1/1 -> Saturation5/1
  Look-Up Table (gear for downshift)/1 -> Rounding Function1/1
  Rounding Function/1 -> Saturation4/1
  Look-Up Table (gear for upshift)/1 -> Rounding Function/1
  "delta speed (\"+\" is acceleration)"/1 -> switch for gear ratio and shifting (muxed)/2, switch for gear number/2
  switch for gear number/1 -> gear number/1
  switch for gear ratio and shifting (muxed)/1 -> gear ratio and shifting/1, New gear ratio/1
  Saturation4/1 -> gear ratio6/1, shifting1/1(gear number), switch for gear number/1
  shifting1/1(out_1) -> Mux/2
  gear ratio6/1 -> Mux/1
  Saturation5/1 -> shifting/1(gear number), gear ratio8/1, total fuel used (gal)/1, switch for gear number/3
  gear ratio8/1 -> Mux2/1
  shifting/1(out_1) -> Mux2/2
  Mux/1 -> switch for gear ratio and shifting (muxed)/1
  Mux2/1 -> switch for gear ratio and shifting (muxed)/3
  prev veh speed/1 -> "delta speed (\"+\" is acceleration)"/1
  "velocity required (limited) "/1 -> Look-Up Table (gear for upshift)/1, Look-Up Table (gear for downshift)/1, "delta speed (\"+\" is acceleration)"/2, prev veh speed/1

== system BD_PAR_AUTO_base_model/<vc> par auto/gearbox control for use w/ AT/allow downshift? ==
  prev gearnum : Inport
  Logical Operator : Logic  Operator=NOR
  Memory : Memory  InitialCondition=1
  Memory1 : Memory  InitialCondition=1
  Relational Operator1 : RelationalOperator  Operator=>  RndMeth=Nearest  InputSameDT=on
  Relational Operator2 : RelationalOperator  Operator=>  RndMeth=Nearest  InputSameDT=on
  allow shift : Outport  InitialOutput=0
  wires:
  Relational Operator2/1 -> Logical Operator/2
  Memory1/1 -> Relational Operator2/2
  Memory/1 -> Memory1/1, Relational Operator1/2
  Relational Operator1/1 -> Logical Operator/1
  prev gearnum/1 -> Relational Operator2/1, Memory/1, Relational Operator1/1
  Logical Operator/1 -> allow shift/1

== system BD_PAR_AUTO_base_model/<vc> par auto/gearbox control for use w/ AT/downshift  command ==
  prev gear number : Inport
  engine load : Inport  Port=2
  engine speed : Inport  Port=3
  Mux : Mux  Inputs=2
  Relational Operator : RelationalOperator  Operator=>  RndMeth=Nearest  InputSameDT=on
  load fraction : Subsystem  mask(Gear Selector){spd=gb_dnshift_spd, load=gb_dnshift_load}
      mask prompts: spd "Speeds:"; load "Load Fractions:"
      mask help:
      | This block will perform a linear interplation (extrapolation outside of bounds) to determine the shift point load fraction associated with the current gear number and speed.
      |
      | The Speeds parameter should be defined as an array of vectors containing speeds for each gear number.  The Load Fractions parameter should be defined as a array of vectors containing load fractions indexed by the speeds in the Speeds parameter for each gear number.
      mask Help:
      | Reference the base workspace variables - gb_**shift_spd and gb_**shift_load  where ** is either up for upshift conditions or dn for downshift conditions.
      | 
      | Or define the arrays as follows:
      | 
      | {[spd1 spd2 spd3 spd4]; [spd1 spd2 spd3 spd4]; ...}
      | 
      | {[load1 load2 load3 load4]; [load1 load2 load3 load4]; ...}
      | 
      | where each array contains one row for each gear in the gearbox.  Speeds should be defined in rad/s and loads as a decimal fraction.
  command : Outport  InitialOutput=0
  wires:
  load fraction/1(Out1) -> Relational Operator/2
  Mux/1 -> load fraction/1(In1)
  engine load/1 -> Relational Operator/1
  prev gear number/1 -> Mux/1
  engine speed/1 -> Mux/2
  Relational Operator/1 -> command/1

== system BD_PAR_AUTO_base_model/<vc> par auto/gearbox control for use w/ AT/downshift  command1 ==
  prev gear number : Inport
  engine load : Inport  Port=2
  engine speed : Inport  Port=3
  Mux : Mux  Inputs=2
  Relational Operator : RelationalOperator  Operator=>  RndMeth=Nearest  InputSameDT=on
  load fraction : Subsystem  mask(Gear Selector){spd=gb_dnshift_spd, load=gb_dnshift_load}
      mask prompts: spd "Speeds:"; load "Load Fractions:"
      mask help:
      | This block will perform a linear interplation (extrapolation outside of bounds) to determine the shift point load fraction associated with the current gear number and speed.
      |
      | The Speeds parameter should be defined as an array of vectors containing speeds for each gear number.  The Load Fractions parameter should be defined as a array of vectors containing load fractions indexed by the speeds in the Speeds parameter for each gear number.
      mask Help:
      | Reference the base workspace variables - gb_**shift_spd and gb_**shift_load  where ** is either up for upshift conditions or dn for downshift conditions.
      | 
      | Or define the arrays as follows:
      | 
      | {[spd1 spd2 spd3 spd4]; [spd1 spd2 spd3 spd4]; ...}
      | 
      | {[load1 load2 load3 load4]; [load1 load2 load3 load4]; ...}
      | 
      | where each array contains one row for each gear in the gearbox.  Speeds should be defined in rad/s and loads as a decimal fraction.
  command : Outport  InitialOutput=0
  wires:
  Relational Operator/1 -> command/1
  prev gear number/1 -> Mux/1
  engine load/1 -> Relational Operator/1
  Mux/1 -> load fraction/1(In1)
  load fraction/1(Out1) -> Relational Operator/2
  engine speed/1 -> Mux/2
